simulink model "vehicle_model_v3"  (R2015a)
settings: Solver=ode3  StartTime=0.0  StopTime=360  FixedStep=1e-1  RelTol=1e-3
values from neighbouring files (symbols this model uses):
  P = zeros(path_length*segment_length,2)    [random_path_generate.m]
  vehicle_length = 5    [setup.m]
undefined symbols (not defined in the file): animation_update_interval, datetime, enable_CG_trace, enable_rearAxle_trace, plotAxisLimitMode, plotAxisLimits, save_anim_frames, vehicle_width
libraries: simulink x1
settings Model: CovModelRefEnable=off  Creator=Prateek Mallya  LastModifiedBy=root
settings DataIOCC: LimitDataPoints=off  SaveFormat=StructureWithTime
settings HardwareCC: ProdBitPerPointer=64  ProdLargestAtomicFloat=Float  ProdIntDivRoundTo=Zero  ProdEndianess=LittleEndian  ProdHWDeviceType=Specified
settings ModelReferenceCC: PropagateSignalLabelsOutOfModel=on

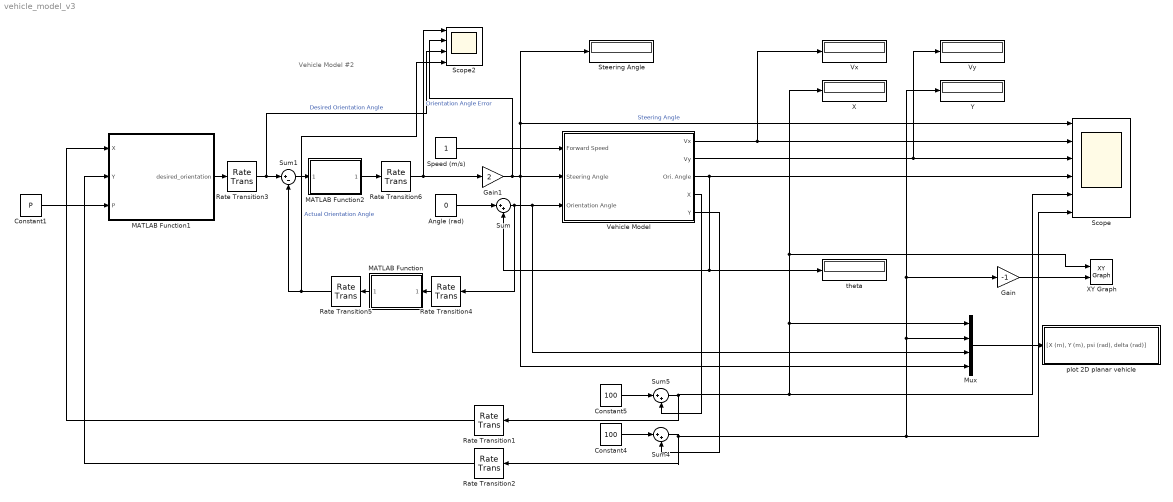
== system vehicle_model_v3 ==
  note: Vehicle Model #2
  Angle (rad) : Constant  Value=0
  Constant1 : Constant  Value=P
  Constant4 : Constant  Value=100
  Constant5 : Constant  Value=100
  Gain : Gain  Gain=-1
  Gain1 : Gain  Gain=2
  MATLAB Function : MATLAB Function  TreatAsAtomicUnit=on
  MATLAB Function1 : MATLAB Function  TreatAsAtomicUnit=on
  MATLAB Function2 : MATLAB Function  TreatAsAtomicUnit=on
  Mux : Mux
  Rate Transition{1..6} (6 alike) : RateTransition
  Scope : Scope  NumInputPorts=6
      settings: YMin=-0.14625~-1.06831~-1.125~-2.88599~13.54446~-133.93215  YMax=0.01625~1.22981~0.125~0.32067~78.0999~14.88135
  Scope2 : Scope  NumInputPorts=4
      settings: YMin=0~-0.35~0~0  YMax=3.5~0~7~1.25  SaveName=ScopeData2
  Speed (m/s) : Constant
  Steering Angle : Display
  Sum : Sum  Inputs=|++
  Sum1 : Sum  Inputs=|+-
  Sum4 : Sum  Inputs=|++
  Sum5 : Sum  Inputs=|++
  Vehicle Model : Subsystem
  Vx : Display
  Vy : Display
  X : Display
  XY Graph : simulink/Sinks/XY Graph  xmin=-60  xmax=180  ymin=-100  ymax=40  st=-1
  Y : Display
  plot 2D planar vehicle : Subsystem  mask(6DoF Animation){axisMode=plotAxisLimitMode, ax=plotAxisLimits, Ts=animation_update_interval, enable_CG_trace=enable_CG_trace, enable_rearAxle_trace=enable_rearAxle_trace, save_anim_frames=save_anim_frames, anim_frame_name_str=char(datetime('now','Format','yyyy-MM-dd_HH_mm_ss')), L=vehicle_length, W=vehicle_width}
      mask prompts: axisMode "Axis Mode (0->auto, 1->fixed, BOTH use Axes Limits below)"; ax "Axes limits [xmin xmax ymin ymax] (m):"; Ts "Time interval between updates (s):"; enable_CG_trace "Enable vehicle CG trace? (0/1)"; enable_rearAxle_trace "Enable rear axle trace? (0/1)"; save_anim_frames "Save animaton frames? (0/1)"; anim_frame_name_str "Animation sequence name (if save frames==1)"; L "Vehicle length (m)"; W "Vehicle width (m)"
      mask help:
      | Create a 2D animated view of a steering vehicle model with tires.
      |
      | Marc Compere
      | CompereM@saic.com
      | created : 22 August 2002
      | modified: 28 Dec 2015
      mask init:
      | Config.axisMode=axisMode;
      | Config.ax=ax;
      | Config.Ts=Ts;
      | Config.enable_CG_trace=enable_CG_trace;
      | Config.enable_rearAxle_trace=enable_rearAxle_trace;
      | Config.save_anim_frames=save_anim_frames;
      | Config.anim_frame_name_str=anim_frame_name_str;
      | Config.L=L;
      | Config.W=W;
      mask Help:
      | <p>This block generates a 3 dimensional display of a simulation trajectory, with the craft orientation displayed during flight</p>
      | 
      | <p>There are two inputs to this block, Position and Euler.  These inputs contain more than one signal as described below.</p>
      | 
      | <p><H4>Block Vector Input - Position</H4>
      | <ul>
      | <li>X Position</li>
      | <li>Y Position</li>
      | <li>Z Position</li>
      | </ul>
      | </p>
      | 
      | <p><H4>Block Vector Input - Euler</H4>
      |     <ul>
      |     <li>Roll Attitude</li>
      |     <li>Pitch Attitude</li>
      |     <li>Yaw Attitude</li>
      |    </ul>
      |    </p>
  theta : Display
  wires:
  Speed (m/s)/1 -> Vehicle Model/1(Forward Speed)
  Angle (rad)/1 -> Sum/1
  Sum/1 -> Rate Transition4/1, Vehicle Model/3(Orientation Angle), Mux/3
  Vehicle Model/1(Vx) -> Scope/2, Vx/1
  Vehicle Model/2(Vy) -> Scope/3, Vy/1
  Vehicle Model/3(Ori. Angle) -> Scope/4, Sum/2, theta/1
  Mux/1 -> plot 2D planar vehicle/1("[X (m), Y (m), psi (rad), delta (rad)]")
  Gain/1 -> XY Graph/2
  Sum1/1 -> MATLAB Function2/1(input_error_angle)
  Constant5/1 -> Sum5/1
  Constant4/1 -> Sum4/1
  Vehicle Model/4(X) -> Sum5/2
  Vehicle Model/5(Y) -> Sum4/2
  Sum5/1 -> Rate Transition1/1, Mux/1, XY Graph/1, X/1, Scope/5
  Sum4/1 -> Rate Transition2/1, Mux/2, Gain/1, Y/1, Scope/6
  MATLAB Function1/1(desired_orientation) -> Rate Transition3/1
  Gain1/1 -> Scope2/2, Mux/4, Scope/1, Steering Angle/1, Vehicle Model/2(Steering Angle)  "Steering Angle"
  Rate Transition1/1 -> MATLAB Function1/1(X)
  Rate Transition2/1 -> MATLAB Function1/2(Y)
  Constant1/1 -> MATLAB Function1/3(P)
  MATLAB Function/1(basic_orientation_angle) -> Rate Transition5/1
  Rate Transition4/1 -> MATLAB Function/1(orientation_angle)
  Rate Transition3/1 -> Scope2/3, Sum1/1  "Desired Orientation Angle"
  MATLAB Function2/1(output_error_angle) -> Rate Transition6/1
  Rate Transition6/1 -> Scope2/1, Gain1/1  "Orientation Angle Error"
  Rate Transition5/1 -> Scope2/4, Sum1/2  "Actual Orientation Angle"

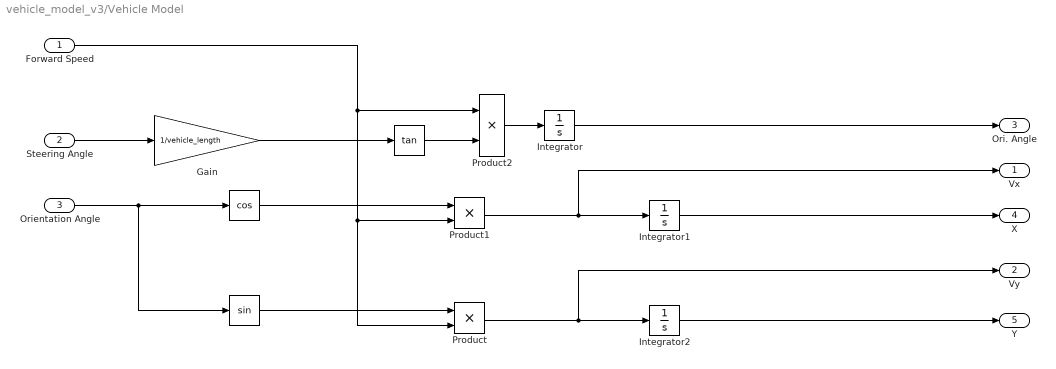
== system vehicle_model_v3/Vehicle Model ==
  Forward Speed : Inport
  Steering Angle : Inport  Port=2
  Orientation Angle : Inport  Port=3
  " " : Trigonometry  Operator=cos
  "  " : Trigonometry
  "    " : Trigonometry  Operator=tan
  Gain : Gain  Gain=1/vehicle_length
  Integrator : Integrator
  Integrator1 : Integrator
  Integrator2 : Integrator
  Product : Product
  Product1 : Product
  Product2 : Product
  Vx : Outport
  Vy : Outport  Port=2
  Ori. Angle : Outport  Port=3
  X : Outport  Port=4
  Y : Outport  Port=5
  wires:
  Steering Angle/1 -> Gain/1
  Orientation Angle/1 -> "  "/1, " "/1
  " "/1 -> Product1/1
  "  "/1 -> Product/1
  Forward Speed/1 -> Product1/2, Product/2, Product2/1
  Gain/1 -> "    "/1
  Integrator/1 -> Ori. Angle/1
  Product/1 -> Vy/1, Integrator2/1
  Product1/1 -> Vx/1, Integrator1/1
  Integrator1/1 -> X/1
  Integrator2/1 -> Y/1
  Product2/1 -> Integrator/1
  "    "/1 -> Product2/2

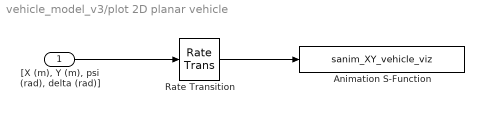
== system vehicle_model_v3/plot 2D planar vehicle ==
  "[X (m), Y (m), psi (rad), delta (rad)]" : Inport
  Animation S-Function : S-Function  FunctionName=sanim_XY_vehicle_viz  Parameters=Config
  Rate Transition : RateTransition  Integrity=off
  wires:
  "[X (m), Y (m), psi (rad), delta (rad)]"/1 -> Rate Transition/1
  Rate Transition/1 -> Animation S-Function/1

== matlab function vehicle_model_v3/MATLAB Function1 ==
  data: X input; desired_orientation output; Y input; P input
function desired_orientation = calculate_desired_orientation(X,Y,P)

look_ahead_distance = 3;

current_position = [Y,X];

[closest,closest_index] = find_closest_path_coordinate(P,current_position);

desired_vector_head_point = P(closest_index + look_ahead_distance,:);
desired_vector_tail_point = current_position;

desired_orientation = find_angle(desired_vector_head_point,desired_vector_tail_point);

% desired_vector_head_point
% desired_vector_tail_point
% desired_orientation

end

== matlab function vehicle_model_v3/MATLAB Function ==
  data: orientation_angle input; basic_orientation_angle output
function basic_orientation_angle = get_basic_orientation_angle(orientation_angle)

if orientation_angle < 0
    while orientation_angle<0
        orientation_angle = orientation_angle + 2*pi;
    end
elseif orientation_angle >= 2*pi
    while orientation_angle>=2*pi
        orientation_angle = orientation_angle - 2*pi;
    end
end
basic_orientation_angle = orientation_angle;
end

== matlab function vehicle_model_v3/MATLAB Function2 ==
  data: input_error_angle input; output_error_angle output
function output_error_angle = angle_error_correction(input_error_angle)
%output_error_angle = input_error_angle;
if input_error_angle<-pi
    output_error_angle =  input_error_angle + 2*pi;
elseif input_error_angle>pi
    output_error_angle = input_error_angle - 2*pi;
else
    output_error_angle = input_error_angle;
end

end
